simulink model "heat_exchanger_2DOFPID"  (R2017b)
settings: Solver=VariableStepAuto  StartTime=0.0  StopTime=500  RelTol=1e-3
values from neighbouring files (symbols this model uses):
  Area = n*A_heat_plate    (= 9.8716)    [heat_exchanger_config.m]    (also in linearization.m = 20)
  cp_H2O = 4190    [heat_exchanger_config.m]    (also in linearization.m)
  cp_wort = 4062    [heat_exchanger_config.m]    (also in linearization.m = 4000)
  HE_delay = 25    [heat_exchanger_config.m]    (also in linearization.m = 5)
  m_H2O = m_wort    (= 10)    [heat_exchanger_config.m]    (also in linearization.m = 1)
  m_wort = 10    [heat_exchanger_config.m]    (also in linearization.m = 1)
  rho_wort = 1.06    [heat_exchanger_config.m]    (also in linearization.m)
  T_H2O_in = 5    [heat_exchanger_config.m]    (also in linearization.m = 10)
  T_wort_in = 95    [heat_exchanger_config.m]    (also in linearization.m = 70)
  U = (m_dot_h_data*cp_wort*(T_wort_in-T_wort_out)*log(Delta_T2/Delta_T1))/     (Area*(Delta_T2-Delta_T1))    [heat_exchanger_config.m]    (also in linearization.m = 1000)
libraries: simulink x4
settings Model: Creator=Alexander  LastModifiedBy=Oscar

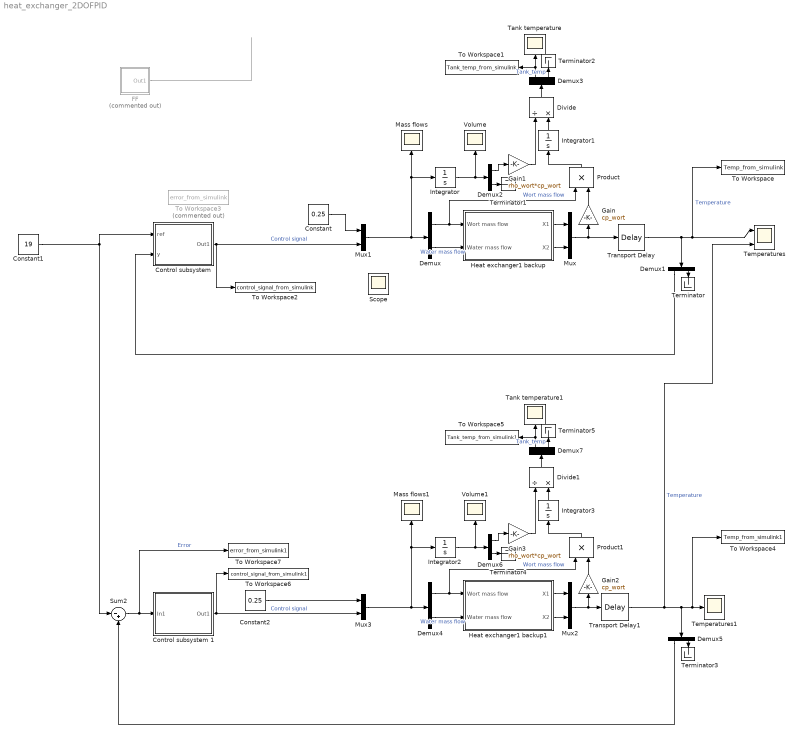
== system heat_exchanger_2DOFPID ==
  Constant : Constant  Value=0.25
  Constant1 : Constant  Value=19
  Constant2 : Constant  Value=0.25
  "Control subsystem " : Subsystem
  Control subsystem 1 : Subsystem
  Demux{,1..7} (8 alike) : Demux  Outputs=2
  Divide : Product  Inputs=/*
  Divide1 : Product  Inputs=/*
  FF : Subsystem  Commented=on
  Gain : Gain  Gain=cp_wort
  Gain1 : Gain  Gain=rho_wort*cp_wort
  Gain2 : Gain  Gain=cp_wort
  Gain3 : Gain  Gain=rho_wort*cp_wort
  Heat exchanger1 backup : Subsystem
  Heat exchanger1 backup1 : Subsystem
  Integrator{,1..3} (4 alike) : Integrator
  Mass flows : Scope
  Mass flows1 : Scope
  Mux{,1..3} (4 alike) : Mux  Inputs=2
  Product : Product
  Product1 : Product
  Scope : Scope
  Sum2 : Sum  Inputs=|-+
  Tank temperature : Scope
  Tank temperature1 : Scope
  Temperatures : Scope  NumInputPorts=2
  Temperatures1 : Scope
  Terminator{,1..5} (6 alike) : Terminator
  To Workspace : ToWorkspace  VariableName=Temp_from_simulink  SaveFormat=Timeseries  SampleTime=-1
  To Workspace1 : ToWorkspace  VariableName=Tank_temp_from_simulink  SaveFormat=Timeseries  SampleTime=-1
  To Workspace2 : ToWorkspace  VariableName=control_signal_from_simulink  SaveFormat=Timeseries  SampleTime=-1
  To Workspace3 : ToWorkspace  Commented=on  VariableName=error_from_simulink  SaveFormat=Timeseries  SampleTime=-1
  To Workspace4 : ToWorkspace  VariableName=Temp_from_simulink1  SaveFormat=Timeseries  SampleTime=-1
  To Workspace5 : ToWorkspace  VariableName=Tank_temp_from_simulink1  SaveFormat=Timeseries  SampleTime=-1
  To Workspace6 : ToWorkspace  VariableName=control_signal_from_simulink1  SaveFormat=Timeseries  SampleTime=-1
  To Workspace7 : ToWorkspace  VariableName=error_from_simulink1  SaveFormat=Timeseries  SampleTime=-1
  Transport Delay : TransportDelay  DelayTime=HE_delay
  Transport Delay1 : TransportDelay  DelayTime=HE_delay
  Volume : Scope
  Volume1 : Scope
  wires:
  Demux/2 -> Heat exchanger1 backup/2(Water mass flow)  "Water mass flow"
  Demux/1 -> Product/1, Heat exchanger1 backup/1(Wort mass flow)  "Wort mass flow"
  Mux/1 -> Gain/1, Transport Delay/1
  Integrator/1 -> Demux2/1, Volume/1
  Transport Delay/1 -> Demux1/1, To Workspace/1, Temperatures/1  "Temperature"
  Demux1/2 -> Terminator/1
  Mux1/1 -> Integrator/1, Mass flows/1, Demux/1
  Constant/1 -> Mux1/1
  Demux1/1 -> "Control subsystem "/2(y)
  Heat exchanger1 backup/1(X1) -> Mux/1
  Heat exchanger1 backup/2(X2) -> Mux/2
  Integrator1/1 -> Divide/2
  Gain1/1 -> Divide/1
  Product/1 -> Integrator1/1
  Gain/1 -> Product/2
  Demux2/1 -> Gain1/1
  Demux2/2 -> Terminator1/1
  Demux3/2 -> Terminator2/1
  Divide/1 -> Demux3/1
  Demux3/1 -> Tank temperature/1, To Workspace1/1  "Tank_temp"
  Constant1/1 -> "Control subsystem "/1(ref), Sum2/1
  "Control subsystem "/1(Out1) -> Mux1/2, To Workspace2/1  "Control signal"
  Gain2/1 -> Product1/2
  Demux5/2 -> Terminator3/1
  Demux6/2 -> Terminator4/1
  Mux2/1 -> Gain2/1, Transport Delay1/1
  Demux7/1 -> Tank temperature1/1, To Workspace5/1  "Tank_temp"
  Divide1/1 -> Demux7/1
  Sum2/1 -> To Workspace7/1, Control subsystem 1/1(In1)  "Error"
  Demux7/2 -> Terminator5/1
  Demux5/1 -> Sum2/2
  Constant2/1 -> Mux3/1
  Heat exchanger1 backup1/1(X1) -> Mux2/1
  Demux6/1 -> Gain3/1
  Demux4/2 -> Heat exchanger1 backup1/2(Water mass flow)  "Water mass flow"
  Product1/1 -> Integrator3/1
  Control subsystem 1/1(Out1) -> Mux3/2, To Workspace6/1  "Control signal"
  Integrator2/1 -> Demux6/1, Volume1/1
  Transport Delay1/1 -> Temperatures/2, Demux5/1, To Workspace4/1, Temperatures1/1  "Temperature"
  Gain3/1 -> Divide1/1
  Demux4/1 -> Product1/1, Heat exchanger1 backup1/1(Wort mass flow)  "Wort mass flow"
  Heat exchanger1 backup1/2(X2) -> Mux2/2
  Integrator3/1 -> Divide1/2
  Mux3/1 -> Integrator2/1, Mass flows1/1, Demux4/1
  FF/1(Out1) -> ?

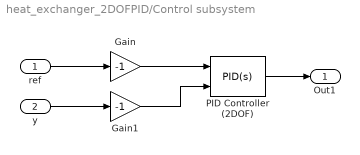
== system heat_exchanger_2DOFPID/Control subsystem  ==
  ref : Inport
  y : Inport  Port=2
  Gain : Gain  Gain=-1
  Gain1 : Gain  Gain=-1
  PID Controller (2DOF) : simulink/Continuous/PID Controller (2DOF)  Controller=PID  TimeDomain=Continuous-time  SampleTime=-1  IntegratorMethod=Forward Euler  FilterMethod=Forward Euler  Form=Parallel  UseFilter=on  ControllerParametersSource=internal  P=0.015  I=0.0003  D=0  N=100  b=0.5  c=0.005  InitialConditionSource=internal  InitialConditionForIntegrator=0  InitialConditionForFilter=0  ExternalReset=none  LimitOutput=off  UpperSaturationLimit=inf  LowerSaturationLimit=-inf  LinearizeAsGain=on  AntiWindupMode=none  Kb=1  TrackingMode=off  Kt=1  PParamMin=[]  PParamMax=[]  IParamMin=[]  IParamMax=[]  DParamMin=[]  DParamMax=[]  NParamMin=[]  NParamMax=[]  bParamMin=[]  bParamMax=[]  cParamMin=[]  cParamMax=[]  KbParamMin=[]  KbParamMax=[]  KtParamMin=[]  KtParamMax=[]  POutMin=[]  POutMax=[]  IOutMin=[]  IOutMax=[]  DOutMin=[]  DOutMax=[]  NOutMin=[]  NOutMax=[]  bOutMin=[]  bOutMax=[]  cOutMin=[]  cOutMax=[]  KbOutMin=[]  KbOutMax=[]  KtOutMin=[]  KtOutMax=[]  IntegratorOutMin=[]  IntegratorOutMax=[]  FilterOutMin=[]  FilterOutMax=[]  SumOutMin=[]  SumOutMax=[]  Sum1OutMin=[]  Sum1OutMax=[]  Sum2OutMin=[]  Sum2OutMax=[]  Sum3OutMin=[]  Sum3OutMax=[]  SumI1OutMin=[]  SumI1OutMax=[]  SumI2OutMin=[]  SumI2OutMax=[]  SumI3OutMin=[]  SumI3OutMax=[]  SumDOutMin=[]  SumDOutMax=[]  SaturationOutMin=[]  SaturationOutMax=[]  IntegratorContinuousStateAttributes=''  IntegratorStateMustResolveToSignalObject=off  IntegratorRTWStateStorageClass=Auto  FilterContinuousStateAttributes=''  FilterStateMustResolveToSignalObject=off  FilterRTWStateStorageClass=Auto  DifferentiatorICPrevScaledInput=0  DifferentiatorOutMin=[]  DifferentiatorOutMax=[]  InitialConditionSetting=State (most efficient)  FilterDiffOutCoefMin=[]  FilterDiffOutCoefMax=[]  SumDenOutMin=[]  SumDenOutMax=[]  SumNumOutMin=[]  SumNumOutMax=[]  ReciprocalOutMin=[]  ReciprocalOutMax=[]  DivideOutMin=[]  DivideOutMax=[]  TunerSelectOption=Transfer Function Based (PID Tuner App)
  Out1 : Outport
  wires:
  ref/1 -> Gain/1
  y/1 -> Gain1/1
  PID Controller (2DOF)/1 -> Out1/1
  Gain/1 -> PID Controller (2DOF)/1
  Gain1/1 -> PID Controller (2DOF)/2

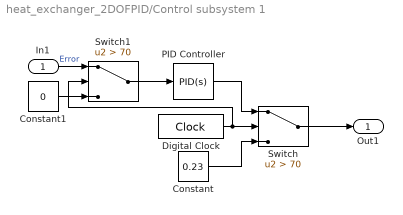
== system heat_exchanger_2DOFPID/Control subsystem 1 ==
  In1 : Inport
  Constant : Constant  Value=0.23
  Constant1 : Constant  Value=0
  Digital Clock : DigitalClock
  PID Controller : simulink/Continuous/PID Controller  Controller=PID  TimeDomain=Continuous-time  SampleTime=-1  IntegratorMethod=Forward Euler  FilterMethod=Forward Euler  Form=Parallel  UseFilter=on  ControllerParametersSource=internal  P=0.01  I=0.0001  D=0  N=100  InitialConditionSource=internal  InitialConditionForIntegrator=0  InitialConditionForFilter=0  ExternalReset=none  LimitOutput=on  UpperSaturationLimit=0.5  LowerSaturationLimit=0.1  LinearizeAsGain=on  AntiWindupMode=back-calculation  Kb=1  TrackingMode=off  Kt=1  PParamMin=[]  PParamMax=[]  IParamMin=[]  IParamMax=[]  DParamMin=[]  DParamMax=[]  NParamMin=[]  NParamMax=[]  KbParamMin=[]  KbParamMax=[]  KtParamMin=[]  KtParamMax=[]  POutMin=[]  POutMax=[]  IOutMin=[]  IOutMax=[]  DOutMin=[]  DOutMax=[]  NOutMin=[]  NOutMax=[]  KbOutMin=[]  KbOutMax=[]  KtOutMin=[]  KtOutMax=[]  IntegratorOutMin=[]  IntegratorOutMax=[]  FilterOutMin=[]  FilterOutMax=[]  SumOutMin=[]  SumOutMax=[]  SumI1OutMin=[]  SumI1OutMax=[]  SumI2OutMin=[]  SumI2OutMax=[]  SumI3OutMin=[]  SumI3OutMax=[]  SumDOutMin=[]  SumDOutMax=[]  SaturationOutMin=[]  SaturationOutMax=[]  IntegratorContinuousStateAttributes=''  IntegratorStateMustResolveToSignalObject=off  IntegratorRTWStateStorageClass=Auto  FilterContinuousStateAttributes=''  FilterStateMustResolveToSignalObject=off  FilterRTWStateStorageClass=Auto  DifferentiatorICPrevScaledInput=0  DifferentiatorOutMin=[]  DifferentiatorOutMax=[]  InitialConditionSetting=State (most efficient)  FilterDiffOutCoefMin=[]  FilterDiffOutCoefMax=[]  SumDenOutMin=[]  SumDenOutMax=[]  SumNumOutMin=[]  SumNumOutMax=[]  ReciprocalOutMin=[]  ReciprocalOutMax=[]  DivideOutMin=[]  DivideOutMax=[]  TunerSelectOption=Transfer Function Based (PID Tuner App)
  Switch : Switch  Criteria=u2 > Threshold  Threshold=70
  Switch1 : Switch  Criteria=u2 > Threshold  Threshold=70
  Out1 : Outport
  wires:
  Digital Clock/1 -> Switch1/2, Switch/2
  Constant/1 -> Switch/3
  PID Controller/1 -> Switch/1
  Switch/1 -> Out1/1
  Switch1/1 -> PID Controller/1
  In1/1 -> Switch1/1  "Error"
  Constant1/1 -> Switch1/3

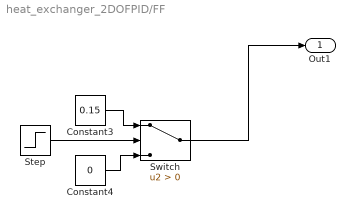
== system heat_exchanger_2DOFPID/FF ==
  Constant3 : Constant  Value=0.15
  Constant4 : Constant  Value=0
  Step : Step  Time=75  SampleTime=0
  Switch : Switch  Criteria=u2 > Threshold
  Out1 : Outport
  wires:
  Constant3/1 -> Switch/1
  Switch/1 -> Out1/1
  Constant4/1 -> Switch/3
  Step/1 -> Switch/2

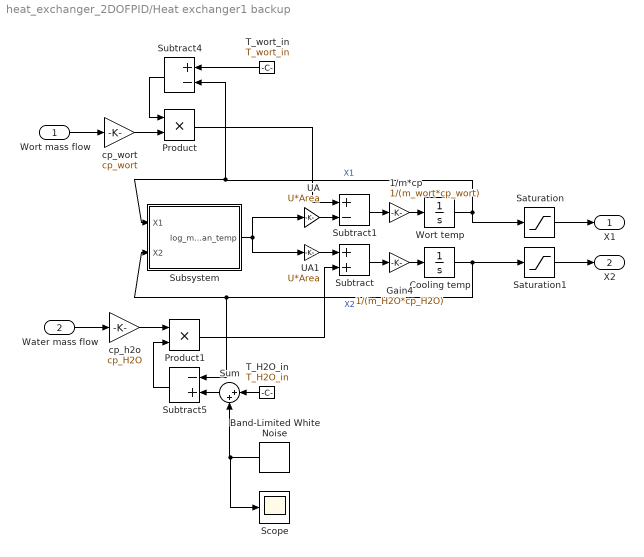
== system heat_exchanger_2DOFPID/Heat exchanger1 backup ==
  Wort mass flow : Inport
  Water mass flow : Inport  Port=2
  "1/m*cp " : Gain  Gain=1/(m_wort*cp_wort)
  Band-Limited White Noise : simulink/Sources/Band-Limited White Noise  Cov=[5]  Ts=100  seed=[23341]
  Cooling temp : Integrator  InitialCondition=T_H2O_in-0.1
  Gain4 : Gain  Gain=1/(m_H2O*cp_H2O)
  Product : Product
  Product1 : Product
  Saturation : Saturate  UpperLimit=T_wort_in  LowerLimit=T_H2O_in
  Saturation1 : Saturate  UpperLimit=T_wort_in  LowerLimit=T_H2O_in
  Scope : Scope
  Subsystem : Subsystem
  Subtract : Sum
  Subtract1 : Sum  Inputs=+-
  Subtract4 : Sum  Inputs=+-
  Subtract5 : Sum  Inputs=-+
  Sum : Sum  Inputs=|++
  T_H2O_in : Constant  Value=T_H2O_in
  T_wort_in : Constant  Value=T_wort_in
  UA : Gain  Gain=U*Area
  "UA1 " : Gain  Gain=U*Area
  Wort temp : Integrator  InitialCondition=T_wort_in-0.1
  cp_h2o : Gain  Gain=cp_H2O
  cp_wort : Gain  Gain=cp_wort
  X1 : Outport
  X2 : Outport  Port=2
  wires:
  Cooling temp/1 -> Saturation1/1, Subtract5/1, Subsystem/2(X2)  "X2"
  "1/m*cp "/1 -> Wort temp/1
  Wort temp/1 -> Saturation/1, Subsystem/1("X1 "), Subtract4/2  "X1"
  UA/1 -> Subtract1/2
  Subtract1/1 -> "1/m*cp "/1
  Gain4/1 -> Cooling temp/1
  "UA1 "/1 -> Subtract/1
  Subtract/1 -> Gain4/1
  T_wort_in/1 -> Subtract4/1
  Subtract5/1 -> Product1/2
  Product/1 -> Subtract1/1
  Subtract4/1 -> Product/1
  Water mass flow/1 -> cp_h2o/1
  Wort mass flow/1 -> cp_wort/1
  Product1/1 -> Subtract/2
  cp_h2o/1 -> Product1/1
  cp_wort/1 -> Product/2
  Subsystem/1(log_mean_temp) -> UA/1, "UA1 "/1
  Saturation/1 -> X1/1
  Saturation1/1 -> X2/1
  Sum/1 -> Subtract5/2
  T_H2O_in/1 -> Sum/1
  Band-Limited White Noise/1 -> Scope/1, Sum/2

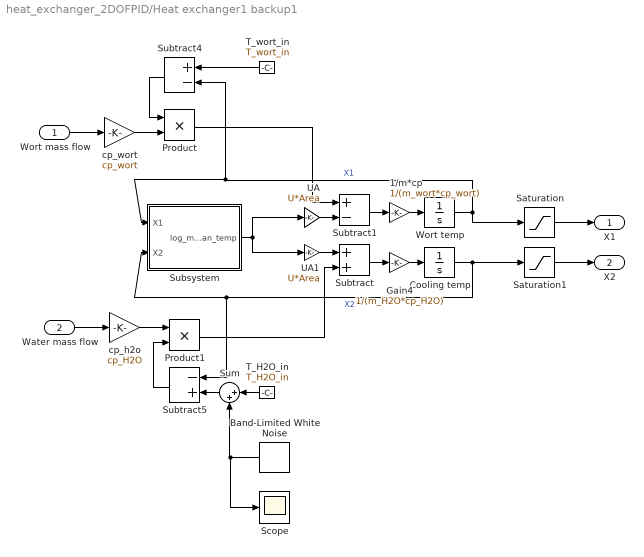
== system heat_exchanger_2DOFPID/Heat exchanger1 backup1 ==
  Wort mass flow : Inport
  Water mass flow : Inport  Port=2
  "1/m*cp " : Gain  Gain=1/(m_wort*cp_wort)
  Band-Limited White Noise : simulink/Sources/Band-Limited White Noise  Cov=[5]  Ts=100  seed=[23341]
  Cooling temp : Integrator  InitialCondition=T_H2O_in-0.1
  Gain4 : Gain  Gain=1/(m_H2O*cp_H2O)
  Product : Product
  Product1 : Product
  Saturation : Saturate  UpperLimit=T_wort_in  LowerLimit=T_H2O_in
  Saturation1 : Saturate  UpperLimit=T_wort_in  LowerLimit=T_H2O_in
  Scope : Scope
  Subsystem : Subsystem
  Subtract : Sum
  Subtract1 : Sum  Inputs=+-
  Subtract4 : Sum  Inputs=+-
  Subtract5 : Sum  Inputs=-+
  Sum : Sum  Inputs=|++
  T_H2O_in : Constant  Value=T_H2O_in
  T_wort_in : Constant  Value=T_wort_in
  UA : Gain  Gain=U*Area
  "UA1 " : Gain  Gain=U*Area
  Wort temp : Integrator  InitialCondition=T_wort_in-0.1
  cp_h2o : Gain  Gain=cp_H2O
  cp_wort : Gain  Gain=cp_wort
  X1 : Outport
  X2 : Outport  Port=2
  wires:
  Cooling temp/1 -> Saturation1/1, Subtract5/1, Subsystem/2(X2)  "X2"
  "1/m*cp "/1 -> Wort temp/1
  Wort temp/1 -> Saturation/1, Subsystem/1("X1 "), Subtract4/2  "X1"
  UA/1 -> Subtract1/2
  Subtract1/1 -> "1/m*cp "/1
  Gain4/1 -> Cooling temp/1
  "UA1 "/1 -> Subtract/1
  Subtract/1 -> Gain4/1
  T_wort_in/1 -> Subtract4/1
  Subtract5/1 -> Product1/2
  Product/1 -> Subtract1/1
  Subtract4/1 -> Product/1
  Water mass flow/1 -> cp_h2o/1
  Wort mass flow/1 -> cp_wort/1
  Product1/1 -> Subtract/2
  cp_h2o/1 -> Product1/1
  cp_wort/1 -> Product/2
  Subsystem/1(log_mean_temp) -> UA/1, "UA1 "/1
  Saturation/1 -> X1/1
  Saturation1/1 -> X2/1
  Sum/1 -> Subtract5/2
  T_H2O_in/1 -> Sum/1
  Band-Limited White Noise/1 -> Scope/1, Sum/2

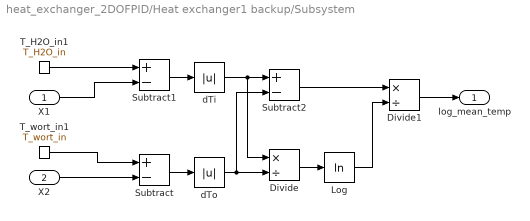
== system heat_exchanger_2DOFPID/Heat exchanger1 backup/Subsystem ==
  "X1 " : Inport
  X2 : Inport  Port=2
  Divide : Product  Inputs=*/
  Divide1 : Product  Inputs=*/
  Log : Math  Operator=log  SaturateOnIntegerOverflow=on
  Subtract : Sum  Inputs=+-
  Subtract1 : Sum  Inputs=+-
  Subtract2 : Sum  Inputs=+-
  T_H2O_in1 : Constant  Value=T_H2O_in
  T_wort_in1 : Constant  Value=T_wort_in
  dTi : Abs
  dTo : Abs
  log_mean_temp : Outport
  wires:
  Subtract/1 -> dTo/1
  T_wort_in1/1 -> Subtract/1
  X2/1 -> Subtract/2
  Subtract1/1 -> dTi/1
  "X1 "/1 -> Subtract1/2
  T_H2O_in1/1 -> Subtract1/1
  dTo/1 -> Subtract2/2, Divide/2
  dTi/1 -> Subtract2/1, Divide/1
  Divide/1 -> Log/1
  Log/1 -> Divide1/2
  Divide1/1 -> log_mean_temp/1
  Subtract2/1 -> Divide1/1

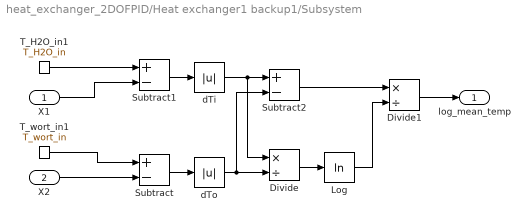
== system heat_exchanger_2DOFPID/Heat exchanger1 backup1/Subsystem ==
  "X1 " : Inport
  X2 : Inport  Port=2
  Divide : Product  Inputs=*/
  Divide1 : Product  Inputs=*/
  Log : Math  Operator=log  SaturateOnIntegerOverflow=on
  Subtract : Sum  Inputs=+-
  Subtract1 : Sum  Inputs=+-
  Subtract2 : Sum  Inputs=+-
  T_H2O_in1 : Constant  Value=T_H2O_in
  T_wort_in1 : Constant  Value=T_wort_in
  dTi : Abs
  dTo : Abs
  log_mean_temp : Outport
  wires:
  Subtract/1 -> dTo/1
  T_wort_in1/1 -> Subtract/1
  X2/1 -> Subtract/2
  Subtract1/1 -> dTi/1
  "X1 "/1 -> Subtract1/2
  T_H2O_in1/1 -> Subtract1/1
  dTo/1 -> Subtract2/2, Divide/2
  dTi/1 -> Subtract2/1, Divide/1
  Divide/1 -> Log/1
  Log/1 -> Divide1/2
  Divide1/1 -> log_mean_temp/1
  Subtract2/1 -> Divide1/1
